simulink model "rtfilter"  (Simulink 6.0)
settings: Solver=ode4  StartTime=0.0  StopTime=10.0  RelTol=1e-3
PostLoadFcn:
  | if ~exist('dsparch4','file') errordlg('Signal Processing Blockset is required to run this demo.', 'Signal Processing Blockset required'); end
libraries: rtwinlib x2, dsparch4 x1
settings Model: Creator=Houska  LastModifiedBy=Houska  ExtModeMexFile=rtwinext  ExtModeTrigType=signal  ProdHWDeviceType=32-bit Real-Time Windows Target
settings ConfigSet: SimulationMode=external
settings DataIOCC: SaveOutput=off  SaveTime=off  SignalLoggingName=logsOut
settings OptimizationCC: MultiInstanced=off
settings FormatCC: IgnoreBidirectionalLines=off
settings HardwareCC: ProdIntDivRoundTo=Zero  ProdEndianess=LittleEndian  ProdHWDeviceType=32-bit Real-Time Windows Target
settings RTWCC: SystemTargetFile=rtwin.tlc  TemplateMakefile=rtwin.tmf  Description=Real-Time Windows Target  ProcessScript=rtwin_make_rtw_hook
settings CodeAppCC: SimulinkBlockComments=off
settings RTWinTargetCC: TargetFcnLib=iso_c_tmw.mat  CCOptimize=on

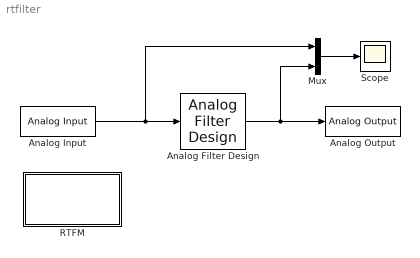
== system rtfilter ==
  Analog Filter Design : dsparch4/Analog Filter Design  method=Butterworth  filttype=Lowpass  N=4  Wlo=500  Whi=80  Rp=3  Rs=40
  Analog Input : rtwinlib/Analog Input  SampleTime=2e-4  DrvAddress=768  DrvOptions=0  Channels=1  RangeMode=1  VoltRange=1
  Analog Output : rtwinlib/Analog Output  SampleTime=2e-4  DrvAddress=0  DrvOptions=0  Channels=1  RangeMode=1  VoltRange=1  InitialValue=[]  FinalValue=[]
  Mux : Mux  Inputs=2
  "RTFM " : Subsystem
      mask Type: Frame-Based Simulation Info
      mask Display: disp('Info')
  Scope : Scope
      settings: TimeRange=0.2  YMin=-1.25659  YMax=1.28483  DataFormat=Structure
  wires:
  Mux/1 -> Scope/1
  Analog Filter Design/1 -> Mux/2, Analog Output/1
  Analog Input/1 -> Mux/1, Analog Filter Design/1

== system rtfilter/RTFM  ==
  note: How to run this demo:
      |
      | 1) Open the Analog Input and Analog Output blocks and select your
      |     data acquisition board.
      |     If there's no board installed, install it using the Install new board button.
      | 2) Build the model using Tools->Real-Time Workshop->Build Model.
      | 3) Connect to the real-time code using Simulation->Connect to target.
      | 4) Start the real-time execution using Simulation->Start real-time code.
      |
      | Note: To run this demo, you must have a data acquisition board plugged into
      | your computer. This demo also requires the Signal Processing Blockset.
